simulink model "EMI_Resilient_Actuator_Phase3"  (R2026a)
settings: Solver=FixedStepDiscrete  StartTime=0  StopTime=1.5  FixedStep=0.001
model workspace (MAT data in the model file):
  EMIPhase3ModelSchema.schema = 'PHASE3-INDEPENDENT-PLANT-V2-31'
  phase3InitialPlantState = [0; 0; 0]
  phase3LoadProfile = [0 0.001 0.002 0.003 0.004 0.005 0.006 0.007 0.008 0.009 0.01 0.011 ... (3002 elements, 1501x2)]
  phase3PlantA = [1  0.000997136251616  0.000228298313718; 0  0.99202969646  0.422222810277; 0  -0.0253333686166  0.612556945724]
  phase3PlantB = [3.16365091086e-05  -0.00332827655811; 0.0913193254874  -6.64757501077; 0.316781256864  0.0913193254874]
  phase3Run : object (value not decoded)
  phase3SampleTime_s = 0.001
Description:
  | Phase 3 integration cross-check: independent discrete actual plant; shared sensor, packet, observer, supervisor and controller logic. This is not an independent implementation of the FDI algorithm.
settings Model: Creator=adand  LastModifiedBy=adand

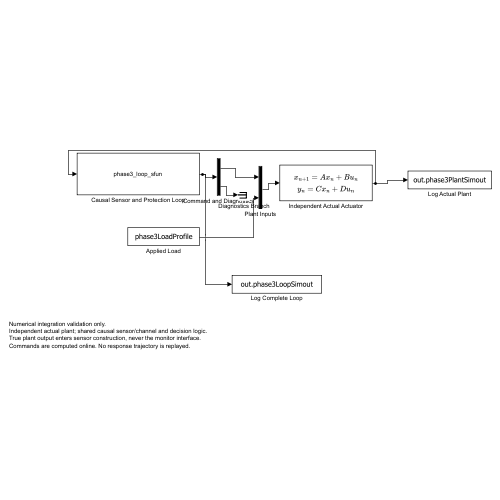
[thumbnail: Simulink's stored preview of the top-level diagram]
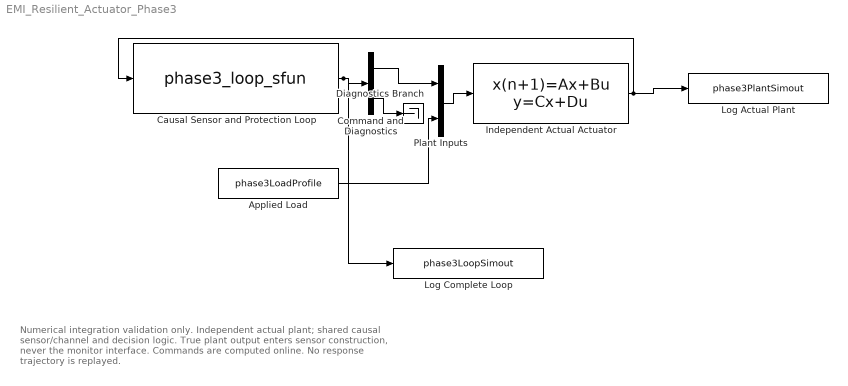
== system EMI_Resilient_Actuator_Phase3 ==
  note: Numerical integration validation only.
      | Independent actual plant; shared causal sensor/channel and decision logic.
      | True plant output enters sensor construction, never the monitor interface.
      | Commands are computed online. No response trajectory is replayed.
  Applied Load : FromWorkspace  VariableName=phase3LoadProfile  SampleTime=phase3SampleTime_s  Interpolate=off  OutputAfterFinalValue=Holding final value
  Causal Sensor and Protection Loop : M-S-Function  FunctionName=phase3_loop_sfun  Parameters=phase3Run
  Command and Diagnostics : Demux  Outputs=[1 30]
  Diagnostics Branch : Terminator
  Independent Actual Actuator : DiscreteStateSpace  A=phase3PlantA  B=phase3PlantB  C=eye(3)  D=zeros(3,2)  InitialCondition=phase3InitialPlantState  SampleTime=phase3SampleTime_s
  Log Actual Plant : ToWorkspace  VariableName=phase3PlantSimout  SaveFormat=Structure With Time  SampleTime=-1
  Log Complete Loop : ToWorkspace  VariableName=phase3LoopSimout  SaveFormat=Structure With Time  SampleTime=-1
  Plant Inputs : Mux  Inputs=2
  wires:
  Independent Actual Actuator/1 -> Causal Sensor and Protection Loop/1, Log Actual Plant/1
  Causal Sensor and Protection Loop/1 -> Command and Diagnostics/1, Log Complete Loop/1
  Command and Diagnostics/1 -> Plant Inputs/1
  Command and Diagnostics/2 -> Diagnostics Branch/1
  Applied Load/1 -> Plant Inputs/2
  Plant Inputs/1 -> Independent Actual Actuator/1
